simulink model "steering_control1"  (R2020b)
settings: Solver=VariableStepAuto  StartTime=0.0  StopTime=10.0  RelTol=1e-3
model workspace (MAT data in the model file):
  ROBOT_L = 0.14
  c = 0
  m = 1
undefined symbols (not defined in the file or in its folder): DiscIntNeverNeededParam
libraries: simulink x1, dspstat3 x1
settings Model: Creator=ped02  LastModifiedBy=ped02

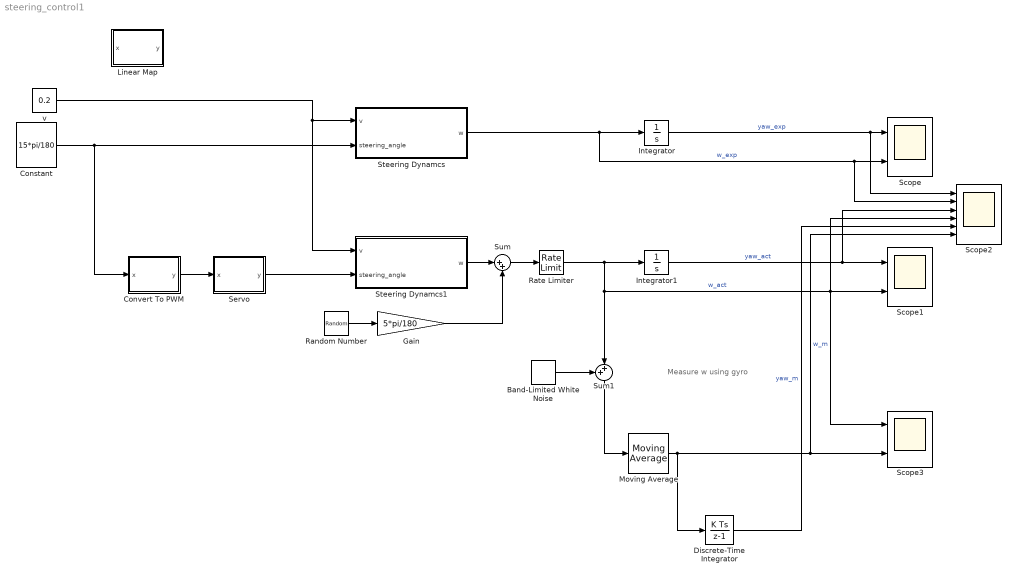
== system steering_control1 ==
  note: Measure w using gyro
  Band-Limited White Noise : simulink/Sources/Band-Limited White Noise  Cov=[0.015]  Ts=0.01  seed=[23341]
  Constant : Constant  Value=15*pi/180
  Convert To PWM : Subsystem  mask{m=-97.7486, c=148}
      mask prompts: m "Gain"; c "Offset"
  Discrete-Time Integrator : DiscreteIntegrator  SampleTime=0.01  ICPrevOutput=DiscIntNeverNeededParam  ICPrevScaledInput=DiscIntNeverNeededParam
  Gain : Gain  Gain=5*pi/180
  Integrator : Integrator
  Integrator1 : Integrator
  Linear Map : Subsystem  mask{m=1, c=0}
      mask prompts: m "Gain"; c "Offset"
  Moving Average : dspstat3/Moving Average  Method=Sliding window  ForgettingFactorPort=off  SpecifyWindowLength=on  WindowLength=16  ForgettingFactor=0.9  SimulateUsing=Code generation
  Random Number : RandomNumber  SampleTime=0.5
  Rate Limiter : RateLimiter  RisingSlewLimit=0.5*2*pi  FallingSlewLimit=-0.5*2*pi  SampleTimeMode=inherited
  Scope : Scope  NumInputPorts=2
  Scope1 : Scope  NumInputPorts=2
  Scope2 : Scope  NumInputPorts=6
  Scope3 : Scope  NumInputPorts=2
  Servo : Subsystem  mask{m=-1/81.576, c=146.3/81.576}
      mask prompts: m "Gain"; c "Offset"
  Steering Dynamcs : Subsystem
  Steering Dynamcs1 : Subsystem
  Sum : Sum  Inputs=|++
  Sum1 : Sum  Inputs=++|
  v : Constant  Value=0.2
  wires:
  Steering Dynamcs/1(w) -> Scope2/2, Scope/2, Integrator/1  "w_exp"
  Integrator/1 -> Scope2/1, Scope/1  "yaw_exp"
  v/1 -> Steering Dynamcs1/1(v), Steering Dynamcs/1(v)
  Constant/1 -> Steering Dynamcs/2(steering_angle), Convert To PWM/1(x)
  Integrator1/1 -> Scope2/3, Scope1/1  "yaw_act"
  Gain/1 -> Sum/2
  Convert To PWM/1(y) -> Servo/1(x)
  Random Number/1 -> Gain/1
  Band-Limited White Noise/1 -> Sum1/1
  Sum1/1 -> Moving Average/1
  Servo/1(y) -> Steering Dynamcs1/2(steering_angle)
  Rate Limiter/1 -> Sum1/2, Scope3/1, Scope2/4, Scope1/2, Integrator1/1  "w_act"
  Steering Dynamcs1/1(w) -> Sum/1
  Sum/1 -> Rate Limiter/1
  Moving Average/1 -> Discrete-Time Integrator/1, Scope3/2, Scope2/6  "w_m"
  Discrete-Time Integrator/1 -> Scope2/5  "yaw_m"

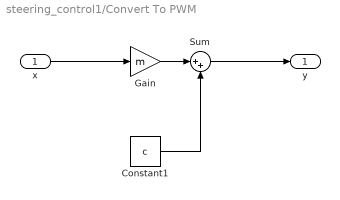
== system steering_control1/Convert To PWM ==
  x : Inport
  Constant1 : Constant  Value=c
  Gain : Gain  Gain=m
  Sum : Sum  Inputs=|++
  y : Outport
  wires:
  Gain/1 -> Sum/1
  Constant1/1 -> Sum/2
  x/1 -> Gain/1
  Sum/1 -> y/1

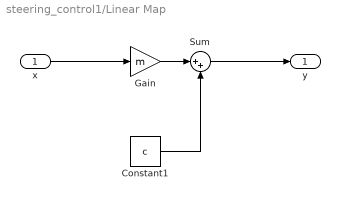
== system steering_control1/Linear Map ==
  x : Inport
  Constant1 : Constant  Value=c
  Gain : Gain  Gain=m
  Sum : Sum  Inputs=|++
  y : Outport
  wires:
  Sum/1 -> y/1
  x/1 -> Gain/1
  Constant1/1 -> Sum/2
  Gain/1 -> Sum/1

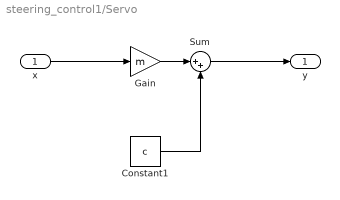
== system steering_control1/Servo ==
  x : Inport
  Constant1 : Constant  Value=c
  Gain : Gain  Gain=m
  Sum : Sum  Inputs=|++
  y : Outport
  wires:
  Sum/1 -> y/1
  x/1 -> Gain/1
  Constant1/1 -> Sum/2
  Gain/1 -> Sum/1

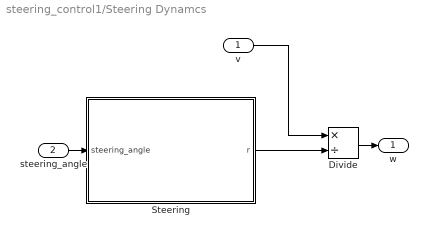
== system steering_control1/Steering Dynamcs ==
  v : Inport
  steering_angle : Inport  Port=2
  Divide : Product  Inputs=*/
  Steering : Subsystem
  w : Outport
  wires:
  steering_angle/1 -> Steering/1(steering_angle)
  Steering/1(r) -> Divide/2
  Divide/1 -> w/1
  v/1 -> Divide/1

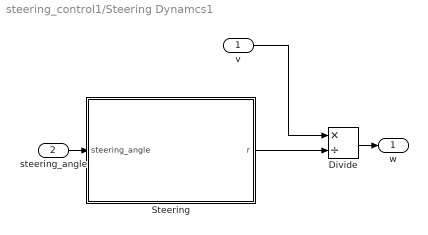
== system steering_control1/Steering Dynamcs1 ==
  v : Inport
  steering_angle : Inport  Port=2
  Divide : Product  Inputs=*/
  Steering : Subsystem
  w : Outport
  wires:
  v/1 -> Divide/1
  Divide/1 -> w/1
  Steering/1(r) -> Divide/2
  steering_angle/1 -> Steering/1(steering_angle)

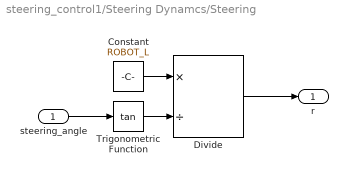
== system steering_control1/Steering Dynamcs/Steering ==
  steering_angle : Inport
  Constant : Constant  Value=ROBOT_L
  Divide : Product  Inputs=*/
  Trigonometric Function : Trigonometry  Operator=tan
  r : Outport
  wires:
  Trigonometric Function/1 -> Divide/2
  steering_angle/1 -> Trigonometric Function/1
  Constant/1 -> Divide/1
  Divide/1 -> r/1

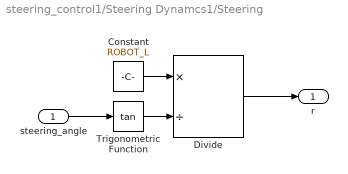
== system steering_control1/Steering Dynamcs1/Steering ==
  steering_angle : Inport
  Constant : Constant  Value=ROBOT_L
  Divide : Product  Inputs=*/
  Trigonometric Function : Trigonometry  Operator=tan
  r : Outport
  wires:
  Divide/1 -> r/1
  Constant/1 -> Divide/1
  steering_angle/1 -> Trigonometric Function/1
  Trigonometric Function/1 -> Divide/2
